simulink subsystem "contactorComLogic"  (R2024b)
settings: Solver=VariableStepAuto  StartTime=0.0  StopTime=10.0  RelTol=1e-3
undefined symbols (not defined in the file): ContactorCmd, DisChrgCmd, DrivetrainEn, DrivetrainEnDelay, PreChrgCmd, VbattMin, VbattThersholdChrg, VbattThresholdDis
settings Model: Creator=E14  LastModifiedBy=E14

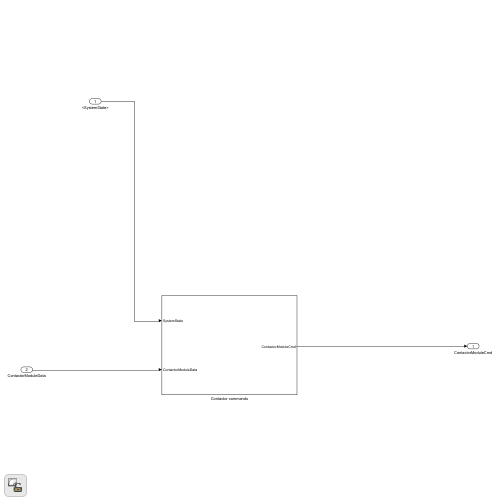
[thumbnail: Simulink's stored preview of the top-level diagram]
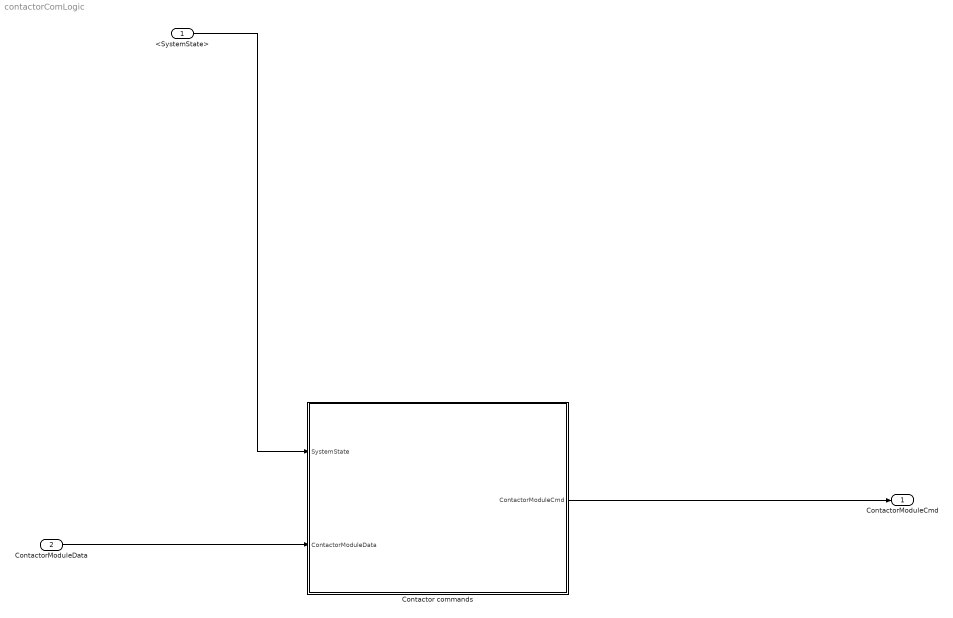
== system contactorComLogic ==
  <SystemState> : Inport
  ContactorModuleData : Inport  Port=2
  Contactor commands : Subsystem
  ContactorModuleCmd : Outport
  wires:
  ContactorModuleData/1 -> Contactor commands/2(ContactorModuleData)
  Contactor commands/1(ContactorModuleCmd) -> ContactorModuleCmd/1
  <SystemState>/1 -> Contactor commands/1(SystemState)

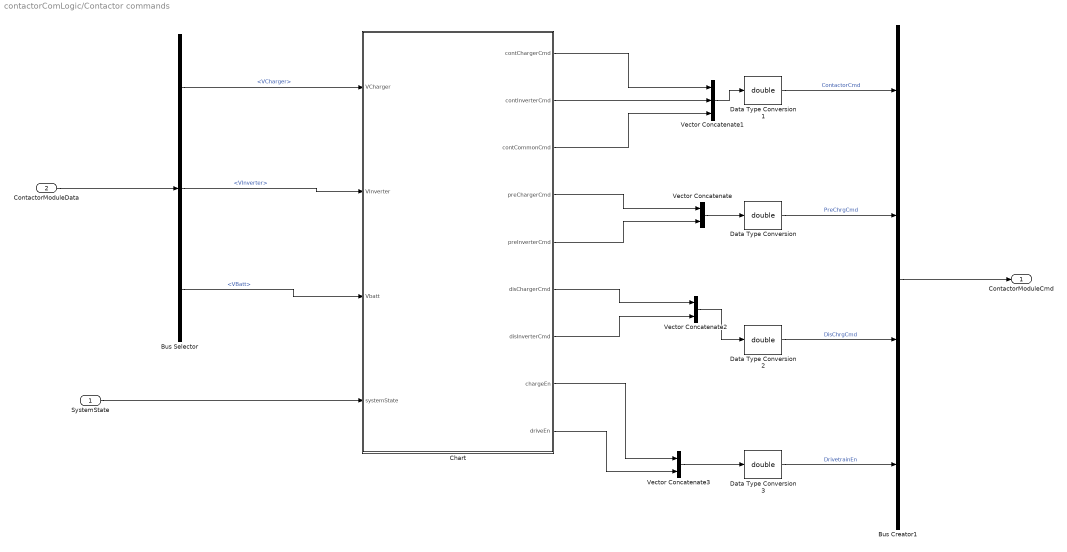
== system contactorComLogic/Contactor commands ==
  SystemState : Inport
  ContactorModuleData : Inport  Port=2
  Bus Creator1 : BusCreator  Inputs=ContactorCmd,PreChrgCmd,DisChrgCmd,DrivetrainEn
  Bus Selector : BusSelector  OutputSignals=VCharger,VInverter,VBatt
  Chart : Stateflow chart  TreatAsAtomicUnit=on
  Data Type Conversion{,1..3} (4 alike) : DataTypeConversion  OutDataTypeStr=double  SaturateOnIntegerOverflow=off  RndMeth=Floor
  Vector Concatenate : Concatenate
  Vector Concatenate1 : Concatenate  NumInputs=3
  Vector Concatenate2 : Concatenate
  Vector Concatenate3 : Concatenate
  ContactorModuleCmd : Outport
  wires:
  Bus Selector/3 -> Chart/3(Vbatt)  "<VBatt>"
  Bus Selector/2 -> Chart/2(VInverter)  "<VInverter>"
  Bus Selector/1 -> Chart/1(VCharger)  "<VCharger>"
  ContactorModuleData/1 -> Bus Selector/1
  Chart/2(contInverterCmd) -> Vector Concatenate1/2
  Bus Creator1/1 -> ContactorModuleCmd/1
  Chart/5(preInverterCmd) -> Vector Concatenate/2
  Chart/1(contChargerCmd) -> Vector Concatenate1/1
  Data Type Conversion1/1 -> Bus Creator1/1  "ContactorCmd"
  Data Type Conversion3/1 -> Bus Creator1/4  "DrivetrainEn"
  Chart/8(chargeEn) -> Vector Concatenate3/1
  SystemState/1 -> Chart/4(systemState)
  Chart/9(driveEn) -> Vector Concatenate3/2
  Vector Concatenate2/1 -> Data Type Conversion2/1
  Chart/6(disChargerCmd) -> Vector Concatenate2/1
  Chart/3(contCommonCmd) -> Vector Concatenate1/3
  Vector Concatenate/1 -> Data Type Conversion/1
  Vector Concatenate3/1 -> Data Type Conversion3/1
  Chart/7(disInverterCmd) -> Vector Concatenate2/2
  Chart/4(preChargerCmd) -> Vector Concatenate/1
  Vector Concatenate1/1 -> Data Type Conversion1/1
  Data Type Conversion/1 -> Bus Creator1/2  "PreChrgCmd"
  Data Type Conversion2/1 -> Bus Creator1/3  "DisChrgCmd"

== stateflow chart contactorComLogic/Contactor commands/Chart ==
  settings: stateMachineType=MOORE_MACHINE
  state en_charger_prechrg
    preChargerCmd = 1;
    contCommonCmd = 1;
  state charging
    preChargerCmd = 0;
    chargeEn = 1;
  state en_charger
    contChargerCmd = 1;
  state dis_charger
    contChargerCmd = 0;
    disChargerCmd = 1;
    chargeEn = 0;
  state init
    contCommonCmd = 0;
    preChargerCmd = 0;
    preInverterCmd = 0;
    contChargerCmd = 0;
    contInverterCmd = 0;
    disChargerCmd = 0;
    disInverterCmd = 0;
    chargeEn = 0;
    driveEn = 0;
  state en_inverter_prechrg
    preInverterCmd = 1;
    contCommonCmd = 1;
  state en_inverter
    contInverterCmd = 1;
  state driving
    preInverterCmd = 0;
    driveEn = 1;
  state dis_inverter
    contInverterCmd = 0;
    disInverterCmd = 1;
    driveEn = 0;
  init -> en_charger_prechrg [order 1] : [(Vbatt > VbattMin) && (systemState==Charging)]
  en_charger_prechrg -> en_charger [order 1] : [VCharger>=VbattThersholdChrg*Vbatt]
  en_charger -> charging : after(DrivetrainEnDelay,sec)
  charging -> dis_charger [order 1] : [systemState ~= Charging]
  charging -> charging [order 2] : [systemState == Charging]
  en_charger_prechrg -> en_charger_prechrg [order 2] : [VCharger < VbattThersholdChrg*Vbatt]
  en_charger_prechrg -> init [order 3] : [systemState~=Driving]
  dis_charger -> init : [VCharger < VbattThresholdDis*Vbatt]
  (default) -> init
  dis_inverter -> init : [VInverter < VbattThresholdDis*Vbatt]
  en_inverter_prechrg -> init [order 3] : [systemState~=Driving]
  init -> en_inverter_prechrg [order 2] : [(Vbatt > VbattMin) && (systemState==Driving)]
  driving -> driving [order 2] : [systemState == Driving]
  en_inverter_prechrg -> en_inverter_prechrg [order 2] : [VInverter < VbattThersholdChrg*Vbatt]
  driving -> dis_inverter [order 1] : [systemState~=Driving]
  en_inverter -> driving : after(DrivetrainEnDelay,sec)
  en_inverter_prechrg -> en_inverter [order 1] : [VInverter>=VbattThersholdChrg*Vbatt]
  data: VCharger input; VInverter input; Vbatt input; systemState input; contChargerCmd output; contInverterCmd output; contCommonCmd output; preChargerCmd output; preInverterCmd output; disChargerCmd output; disInverterCmd output; chargeEn output; driveEn output; VbattThersholdChrg parameter; VbattMin parameter; DrivetrainEnDelay parameter; VbattThresholdDis parameter; Charging local =2; Driving local =1
